simulink model "commdvbt_file"  (R2025b)
settings: Solver=FixedStepDiscrete  StartTime=0.0  StopTime=1  RelTol=1e-3
model workspace (MATLAB code in the model file):
  | commdvbt_tablegen
undefined symbols (not defined in the file or in its folder): EbNodB, M, rsgenpoly, Tsym
libraries: commblkintrlv2 x3, simulink x2, commblkcod2 x1, commchan3 x1, commcnvcod2 x1, commdigbbndam3 x1, commofdm x1, commcnvintrlv2 x1, commrandsrc3 x1
Description:
  | Digital Video Broadcasting - Terrestrial
settings Model: ExtModeTrigMode=oneshot  ExtModeArmWhenConnect=off  ExtModeAutoUpdateStatusClock=off  Creator=The MathWorks, Inc.  LastModifiedBy=mzabiero
settings SolverCC: ZeroCrossControl=DisableAll  AlgebraicLoopSolver=TrustRegion  InsertRTBMode=Auto  MaxZcPerStep=1.0
settings DataIOCC: SaveFormat=Array  SaveOutput=off  SaveTime=off  ReturnWorkspaceOutputs=off  SignalLoggingName=dvbSigsOut
settings OptimizationCC: BlockReduction=off  BooleanDataType=off  OptimizeBlockIOStorage=off  BufferReuse=off  ReuseModelBlockBuffer=off  GlobalBufferReuse=off  ExpressionFolding=off  ExpressionDepthLimit=2147483647.0  LocalBlockOutputs=off  InitFltsAndDblsToZero=on  EfficientMapNaN2IntZero=off  LifeSpan=1  BufferReusableBoundary=off  EfficientTunableParamExpr=on
settings DebuggingCC: SaveWithParameterizedLinksMsg=none  UnderspecifiedInitializationDetection=Classic  MergeDetectMultiDrivingBlocksExec=none  CheckExecutionContextPreStartOutputMsg=on  SignalResolutionControl=TryResolveAllWithWarning  InheritedTsInSrcMsg=none  MultiTaskDSMMsg=warning  MultiTaskCondExecSysMsg=none  SigSpecEnsureSampleTimeMsg=none  FcnCallInpInsideContextMsg=warning  UnconnectedInputMsg=warning  UnconnectedOutputMsg=warning  UnconnectedLineMsg=warning  BusObjectLabelMismatch=none  AllowSymbolicDim=off  StateNameClashWarn=warning  SFUnexpectedBacktrackingDiag=warning  SFNoUnconditionalDefaultTransitionDiag=warning  SFExecutionAtInitializationDiag=none  ArithmeticOperatorsInVariantConditions=warning
settings HardwareCC: ProdBitPerPointer=32.0  ProdBitPerSizeT=32.0  ProdBitPerPtrDiffT=32.0  ProdLargestAtomicFloat=None  ProdIntDivRoundTo=Undefined  ProdEndianess=Unspecified  ProdWordSize=32.0  ProdHWDeviceType=32-bit Generic  TargetBitPerLong=64.0  TargetBitPerPointer=64.0  TargetBitPerSizeT=64.0  TargetBitPerPtrDiffT=64.0  TargetLongLongMode=on  TargetIntDivRoundTo=Zero  TargetEndianess=LittleEndian  TargetWordSize=64.0  TargetHWDeviceType=MATLAB Host
settings ModelReferenceCC: UpdateModelReferenceTargets=IfOutOfDate  EnableRefExpFcnMdlSchedulingChecks=on  PropagateSignalLabelsOutOfModel=off
settings SFSimCC: SimUseLocalCustomCode=off  MATLABDynamicMemAlloc=off  CustomCodeUndefinedFunction=UseInterfaceOnly
settings RTWCC: SystemTargetFile=ert.tlc  TemplateMakefile=ert_default_tmf  RetainRTWFile=on  RTWUseLocalCustomCode=off  GPUComputeCapability=3.5  DLArmComputeVersion=19.05  Description=Real-Time Workshop Embedded Coder (no auto configuration)
settings CodeAppCC: IgnoreCustomStorageClasses=off  CustomSymbolStrType=$N$R$M  StateflowObjectComments=on  InternalIdentifier=Classic
settings ERTTargetCC: InlinedParameterPlacement=Hierarchical  ERTCustomFileTemplate=example_file_process.tlc  ConvertIfToSwitch=off  SuppressUnreachableDefaultCases=off  DynamicArrayContainerType=coder::array  TargetFcnLib=ansi_tfl_tmw.mat  MultiwordLength=2048.0  GenerateSampleERTMain=on  MatFileLogging=on
settings ConfigComp: CovMetricSettings=dw  CovSaveCumulativeToWorkspaceVar=on  CovSaveSingleToWorkspaceVar=on  CovExternalEMLEnable=off  CovSFcnEnable=off

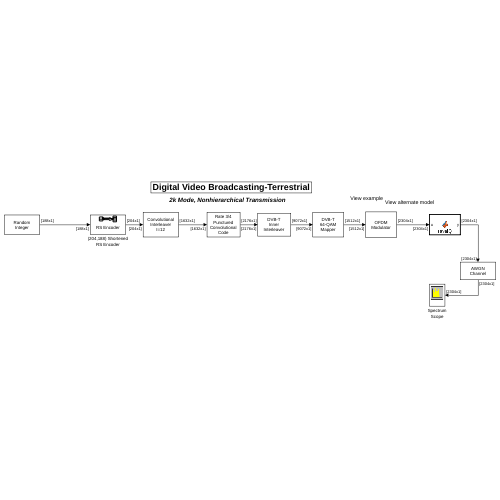
[thumbnail: Simulink's stored preview of the top-level diagram]
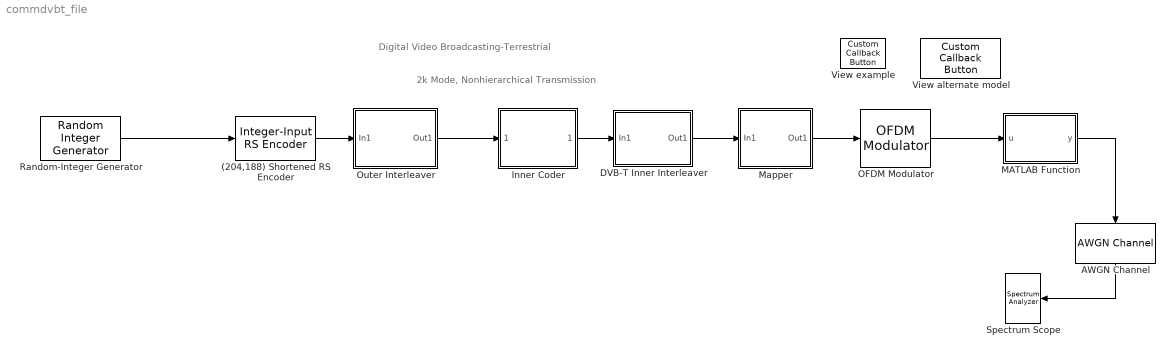
== system commdvbt_file ==
  note: Digital Video Broadcasting-Terrestrial
  note: 2k Mode, Nonhierarchical Transmission
  (204,188) Shortened RS Encoder : commblkcod2/Integer-Input RS Encoder  n=204  k=188  specShortening=off  shortenedK=3  specGenPoly=off  genPoly=rsgenpoly(7,3)  specPrimPoly=off  prPoly=[1 0 1 1]  specPuncture=off  punctVec=[ones(2,1); zeros(2,1)]
  AWGN Channel : commchan3/AWGN Channel  LegacyMode=off  NoiseMethod="Signal to noise ratio  (SNR)"  noiseMode="Signal to noise ratio  (SNR)"  EbNo=10  EsNo=EbNodB+10*log10(log2(M))  SNR=18.5  BitsPerSymbol=1  SignalPower=1/2048  SpecifySymbolPeriod=off  SamplesPerSymbol=round(Tsym / 1.093750e-07)  SymbolPeriod=Tsym  VarianceSource=Parameter  Variance=10^(-0.1*15)/(2048*2)  RandomStream=mt19937ar with seed  Seed=54321  SimulateUsing=Code generation
  DVB-T Inner Interleaver : Subsystem  mask(DVB-T Inner Interleaver){}
      mask init:
      | fullILVec = [(1:126) ...
      |  (rem([0:125]+63,126) +1 + 126     ) ...
      |  (rem([0:125]+105,126)+1 + (2*126) ) ...
      |  (rem([0:125]+42,126) +1 + (3*126) ) ...
      |  (rem([0:125]+21,126) +1 + (4*126) ) ...
      |  (rem([0:125]+84,126) +1 + (5*126) )];
      mask Display: disp('DVB-T\nInner\nInterleaver')
  Inner Coder : Subsystem
      mask Display: disp('Rate 3/4\nPunctured\nConvolutional\nCode');
  MATLAB Function : MATLAB Function  TreatAsAtomicUnit=on
  Mapper : Subsystem  mask(DVB-T 64-QAM Mapper){}
      mask Display: disp('DVB-T\n64-QAM\nMapper')
  OFDM Modulator : commofdm/OFDM Modulator  FFTLength=2048  NumGuardBandCarriers=[268; 268]  InsertDCNull=off  PilotInputPort=off  PilotCarrierIndices=[12; 26; 40; 54]  CyclicPrefixLength=256  Windowing=off  WindowLength=1  OversamplingFactor=1  NumSymbols=1  NumTransmitAntennas=1  SimulateUsing=Interpreted execution
  Outer Interleaver : Subsystem
      mask Display: disp('Convolutional\nInterleaver\nI=12')
  Random-Integer Generator : commrandsrc3/Random Integer Generator  SetSize=256  SeedSource=Parameter  Seed=1234573  SampleTime=Ts % See model workspace  SamplesPerFrame=188  OutputDataType=uint8  SimulateUsing=Interpreted execution
  Spectrum Scope : SpectrumAnalyzer  WindowPosition=[510.000000,324.000000,691.000000,540.000000,]  ScopeFrameLocation=window  SpectrumType=Power density  Method=Welch  SampleRate=9142857.14285714  AxesScaling=Manual  FrequencyResolutionMethod=Window length  WindowLength=2048  FFTLengthSource=Property  FFTLength=2048  Span=10285714.285714285  StartFrequency=-5142857.142857143  StopFrequency=5142857.142857143  AveragingMethod=Running  SpectralAverages=2  SpectrumUnits=dBW/Hz  YLabel=Power spectral density  YLimits=[-140,-90]  AllowFFTLengthLessThanSamplesPerUpdate=on
  View alternate model : CustomCallbackButton  Configuration="{\"components\":[{\"name\":\"BackgroundImageComponent\",\"settings\":{\"image\":{\"size\":[0,0],\"src\":\"default\",\"srcOrientation\":\"Right\"},\"position\":[0,0,1,1]}},{\"name\":\"ButtonStateComponent\",\"settings\":{\"buttonType\":\"momentary\",\"clickFcn\":\"openExample('comm\\/DigitalVideoBroadcastingTerrestrialExample','supportingFile','commdvbt_alt')\",\"onValue\":1,\"position\":[0,0,1,1],\"pressDelay\":\"500\",\"pressFcn\":\"showExample('comm\\/DigitalVideoBroadcastingTerrestrialExample')\",\"repeatInterval\":\"0\",\"states\":[{\"horizontalAlignment\":\"center\",\"image\":{\"position\":[0,0,1,1],\"src\":\"default\",\"srcOrientation\":\"Right\"},\"label\":{\"color\":[0.01176470588,0.01176470588,0.01176470588,1],\"icon\":{\"size\":[0,0],\"src\":\"default\",\"srcOrientation\":\"Right\"},\"iconPlacement\":\"left\",\"text\":{\"content\":\"Alternative version (Demapper computes LLR)\"}},\"labelOffset\":[0,0],\"verticalAlignment\":\"middle\"},{\"horizontalAlignment\":\"center\",\"image\":{\"position\":[0,0,1,1],\"src\":\"default\",\"srcOrientation\":\"Right\"},\"label\":{\"color\":[0.01176470588,0.01176470588,0.01176470588,1],\"icon\":{\"size\":[0,0],\"src\":\"default\",\"srcOrientation\":\"Right\"},\"iconPlacement\":\"left\",\"text\":{\"content\":\"Alternative version (Demapper computes LLR)\"}},\"labelOffset\":[0,0],\"verticalAlignment\":\"middle\"},{\"horizontalAlignment\":\"center\",\"image\":{\"position\":[0,0,1,1],\"src\":\"default\",\"srcOrientation\":\"Right\"},\"label\":{\"color\":[0.01176470588,0.01176470588,0.01176470588,1],\"icon\":{\"size\":[0,0],\"src\":\"default\",\"srcOrientation\":\"Right\"},\"iconPlacement\":\"left\",\"text\":{\"content\":\"Alternative version (Demapper computes LLR)\"}},\"labelOffset\":[0,0],\"verticalAlignment\":\"middle\"},{\"horizontalAlignment\":\"center\",\"image\":{\"position\":[0,0,1,1],\"src\":\"default\",\"srcOrientation\":\"Right\"},\"label\":{\"color\":[0.01176470588,0.01176470588,0.01176470588,1],\"icon\":{\"size\":[0,0],\"src\":\"default\",\"srcOrientation\":\"Right\"},\"iconPlacement\":\"left\",\"text\":{\"content\":\"Alternative version (Demapper computes LLR)\"}},\"labelOffset\":[0,0],\"verticalAlignment\":\"middle\"}]}},{\"name\":\"ForegroundImageComponent\",\"settings\":{\"image\":{\"size\":[0,0],\"src\":\"default\",\"srcOrientation\":\"Right\"},\"isForeground\":1,\"position\":[0,0,1,1]}}],\"derived\":{\"blockParameters\":{\"AutoActivate\":true,\"ButtonText\":\"Alternative version (Demapper computes LLR)\",\"ButtonType\":\"Momentary\",\"ClickFcn\":\"openExample('comm\\/DigitalVideoBroadcastingTerrestrialExample','supportingFile','commdvbt_alt')\",\"OnValue\":1,\"PressDelay\":\"500\",\"PressFcn\":\"showExample('comm\\/DigitalVideoBroadcastingTerrestrialExample')\",\"RepeatInterval\":\"0\",\"fixedAspectRatio\":\"off\"}},\"settings\":{\"BindingType\":\"standalone\",\"autoActivate\":true,\"backgroundColor\":[244,244,244,1],\"backgroundOffset\":0.2,\"backgroundOpacity\":1,\"fixedAspectRatio\":\"off\",\"foregroundColor\":[0.01176470588,0.01176470588,0.01176470588,1],\"migratedFromLegacy\":true,\"useBackgroundColor\":true,\"variant\":\"callback\",\"version\":\"R2025a\"},\"type\":\"Button\"}"  CustomBackgroundColor="{\"color\":[0.9568627451,0.9568627451,0.9568627451],\"show\":true}"
  View example : CustomCallbackButton  Configuration="{\"components\":[{\"name\":\"BackgroundImageComponent\",\"settings\":{\"image\":{\"size\":[0,0],\"src\":\"default\",\"srcOrientation\":\"Right\"},\"position\":[0,0,1,1]}},{\"name\":\"ButtonStateComponent\",\"settings\":{\"buttonType\":\"momentary\",\"clickFcn\":\"showExample('comm\\/DigitalVideoBroadcastingTerrestrialExample')\",\"onValue\":1,\"position\":[0,0,1,1],\"pressDelay\":\"500\",\"pressFcn\":\"showExample('comm\\/DigitalVideoBroadcastingTerrestrialExample')\",\"repeatInterval\":\"0\",\"states\":[{\"horizontalAlignment\":\"center\",\"image\":{\"position\":[0,0,1,1],\"src\":\"default\",\"srcOrientation\":\"Right\"},\"label\":{\"color\":[0.01176470588,0.01176470588,0.01176470588,1],\"icon\":{\"size\":[0,0],\"src\":\"default\",\"srcOrientation\":\"Right\"},\"iconPlacement\":\"left\",\"text\":{\"content\":\"?\"}},\"labelOffset\":[0,0],\"verticalAlignment\":\"middle\"},{\"horizontalAlignment\":\"center\",\"image\":{\"position\":[0,0,1,1],\"src\":\"default\",\"srcOrientation\":\"Right\"},\"label\":{\"color\":[0.01176470588,0.01176470588,0.01176470588,1],\"icon\":{\"size\":[0,0],\"src\":\"default\",\"srcOrientation\":\"Right\"},\"iconPlacement\":\"left\",\"text\":{\"content\":\"?\"}},\"labelOffset\":[0,0],\"verticalAlignment\":\"middle\"},{\"horizontalAlignment\":\"center\",\"image\":{\"position\":[0,0,1,1],\"src\":\"default\",\"srcOrientation\":\"Right\"},\"label\":{\"color\":[0.01176470588,0.01176470588,0.01176470588,1],\"icon\":{\"size\":[0,0],\"src\":\"default\",\"srcOrientation\":\"Right\"},\"iconPlacement\":\"left\",\"text\":{\"content\":\"?\"}},\"labelOffset\":[0,0],\"verticalAlignment\":\"middle\"},{\"horizontalAlignment\":\"center\",\"image\":{\"position\":[0,0,1,1],\"src\":\"default\",\"srcOrientation\":\"Right\"},\"label\":{\"color\":[0.01176470588,0.01176470588,0.01176470588,1],\"icon\":{\"size\":[0,0],\"src\":\"default\",\"srcOrientation\":\"Right\"},\"iconPlacement\":\"left\",\"text\":{\"content\":\"?\"}},\"labelOffset\":[0,0],\"verticalAlignment\":\"middle\"}]}},{\"name\":\"ForegroundImageComponent\",\"settings\":{\"image\":{\"size\":[0,0],\"src\":\"default\",\"srcOrientation\":\"Right\"},\"isForeground\":1,\"position\":[0,0,1,1]}}],\"derived\":{\"blockParameters\":{\"AutoActivate\":true,\"ButtonText\":\"?\",\"ButtonType\":\"Momentary\",\"ClickFcn\":\"showExample('comm\\/DigitalVideoBroadcastingTerrestrialExample')\",\"OnValue\":1,\"PressDelay\":\"500\",\"PressFcn\":\"showExample('comm\\/DigitalVideoBroadcastingTerrestrialExample')\",\"RepeatInterval\":\"0\",\"fixedAspectRatio\":\"off\"}},\"settings\":{\"BindingType\":\"standalone\",\"autoActivate\":true,\"backgroundColor\":[244,244,244,1],\"backgroundOffset\":0.2,\"backgroundOpacity\":1,\"fixedAspectRatio\":\"off\",\"foregroundColor\":[0.01176470588,0.01176470588,0.01176470588,1],\"migratedFromLegacy\":true,\"useBackgroundColor\":true,\"variant\":\"callback\",\"version\":\"R2025a\"},\"type\":\"Button\"}"  CustomBackgroundColor="{\"color\":[0.9568627451,0.9568627451,0.9568627451],\"show\":true}"
  wires:
  Mapper/1(Out1) -> OFDM Modulator/1
  (204,188) Shortened RS Encoder/1 -> Outer Interleaver/1(In1)
  Outer Interleaver/1(Out1) -> Inner Coder/1(Uncoded symbols)
  OFDM Modulator/1 -> MATLAB Function/1(u)
  DVB-T Inner Interleaver/1(Out1) -> Mapper/1(In1)
  Inner Coder/1(Coded bits) -> DVB-T Inner Interleaver/1(In1)
  AWGN Channel/1 -> Spectrum Scope/1
  Random-Integer Generator/1 -> (204,188) Shortened RS Encoder/1
  MATLAB Function/1(y) -> AWGN Channel/1

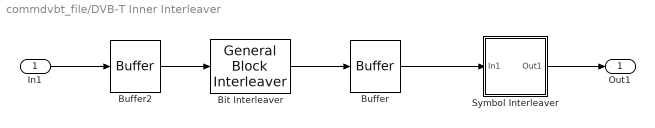
== system commdvbt_file/DVB-T Inner Interleaver ==
  In1 : Inport
  Bit Interleaver : commblkintrlv2/General Block Interleaver  permutationVectorSource=Dialog  elements=dvb_bit_int_table
  Buffer : Buffer  N=9072  OutputFrames=off
  Buffer2 : Buffer  N=756  OutputFrames=off
  Symbol Interleaver : Subsystem
      mask Display:
      | port_label('input', 1, '')
      | port_label('output', 1, '')
      | disp('Symbol\nInterleaver')
  Out1 : Outport
  wires:
  Buffer2/1 -> Bit Interleaver/1
  In1/1 -> Buffer2/1
  Bit Interleaver/1 -> Buffer/1
  Symbol Interleaver/1(Out1) -> Out1/1
  Buffer/1 -> Symbol Interleaver/1(In1)

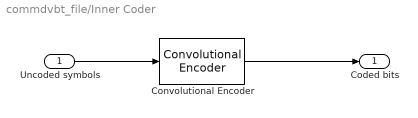
== system commdvbt_file/Inner Coder ==
  Uncoded symbols : Inport
  Convolutional Encoder : commcnvcod2/Convolutional Encoder  trellis=poly2trellis(7, [171 133])  opMode=Continuous  DelayedResetAction=off  hasIniStPort=off  hasFinStPort=off  usePuncVector=on  punctureVector=[1 1 0 1 1 0]'  reset=Unused parameter value
  Coded bits : Outport
  wires:
  Convolutional Encoder/1 -> Coded bits/1
  Uncoded symbols/1 -> Convolutional Encoder/1

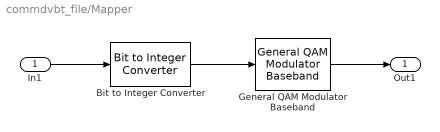
== system commdvbt_file/Mapper ==
  In1 : Inport
  Bit to Integer Converter : simulink/Logic and Bit Operations/Bit to Integer Converter  nbits=6  bitOrder=MSB first  signedOutputValues=Unsigned  outDtype=uint8  outDtypeSigned=Inherit via internal rule
      settings: LibrarySourceBlock=|
      | commutil2/Bit to Integer
      | Converter
  General QAM Modulator Baseband : commdigbbndam3/General QAM Modulator Baseband  SigCon=dvbt_qam  outDtype=double  outWordLen=16  outUDDataType=sfix(16)  outFracLenMode=Best precision  outFracLen=15  outDataTypeStr=double  outLastDataTypeStr=double
  Out1 : Outport
  wires:
  General QAM Modulator Baseband/1 -> Out1/1
  In1/1 -> Bit to Integer Converter/1
  Bit to Integer Converter/1 -> General QAM Modulator Baseband/1

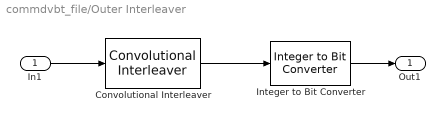
== system commdvbt_file/Outer Interleaver ==
  In1 : Inport
  Convolutional Interleaver : commcnvintrlv2/Convolutional Interleaver  N=12  B=17  ic=0
  Integer to Bit Converter : simulink/Logic and Bit Operations/Integer to Bit Converter  nbits=8  signedInputValues=Unsigned  bitOrder=MSB first  outDtype=boolean
      settings: LibrarySourceBlock=|
      | commutil2/Integer to Bit
      | Converter
  Out1 : Outport
  wires:
  Integer to Bit Converter/1 -> Out1/1
  Convolutional Interleaver/1 -> Integer to Bit Converter/1
  In1/1 -> Convolutional Interleaver/1

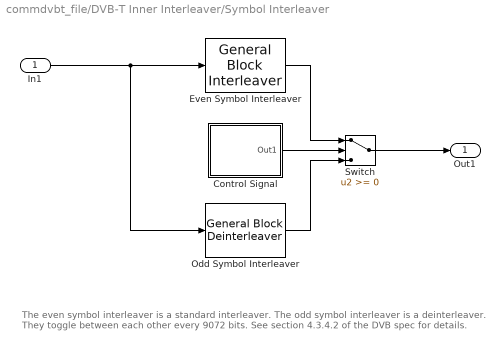
== system commdvbt_file/DVB-T Inner Interleaver/Symbol Interleaver ==
  note: The even symbol interleaver is a standard interleaver.  The odd symbol interleaver is a deinterleaver.  They toggle
      | between each other every 9072 bits.  See section 4.3.4.2 of the DVB spec for details.
  In1 : Inport
  Control Signal : Subsystem
      mask Display:
      | port_label('output', 1, 'ctrl')
      | disp('Control\nSignal')
  Even Symbol Interleaver : commblkintrlv2/General Block Interleaver  permutationVectorSource=Dialog  elements=dvb_sym_int_table
  Odd Symbol Interleaver : commblkintrlv2/General Block Deinterleaver  permutationVectorSource=Dialog  elements=dvb_sym_int_table
  Switch : Switch  SaturateOnIntegerOverflow=off  InputSameDT=off
  Out1 : Outport
  wires:
  In1/1 -> Even Symbol Interleaver/1, Odd Symbol Interleaver/1
  Switch/1 -> Out1/1
  Control Signal/1(Out1) -> Switch/2
  Even Symbol Interleaver/1 -> Switch/1
  Odd Symbol Interleaver/1 -> Switch/3

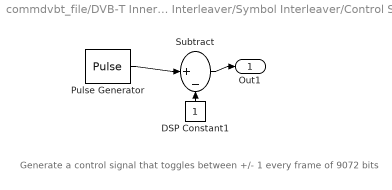
== system commdvbt_file/DVB-T Inner Interleaver/Symbol Interleaver/Control Signal ==
  note: Generate a control signal that toggles between +/- 1 every frame of 9072 bits
  DSP Constant1 : Constant  VectorParams1D=off
  Pulse Generator : DiscretePulseGenerator  Amplitude=2  SampleTime=-1
  Subtract : Sum  Inputs=|+-
  Out1 : Outport
  wires:
  Subtract/1 -> Out1/1
  DSP Constant1/1 -> Subtract/2
  Pulse Generator/1 -> Subtract/1

== matlab function commdvbt_file/MATLAB Function ==
  data: u input; y output
function y = saveIQ(u)
    
    persistent fid
    if isempty(fid)
        folder = '/home/mzabiero/Documents/studia/Inzynierka/data/DVBT_signals';
        filename = fullfile(folder, 'dvbt_sig_sim_iq.dat');
        fid = fopen(filename,'wb');
    end
    
    data = single([real(u(:)).'; imag(u(:)).']);
    data = data(:);
    fwrite(fid, data, 'float32');
    y = u;
end
